simulink model "gm_hybrid_lht"  (R2019b)
settings: Solver=FixedStepDiscrete  StartTime=0.0  StopTime=inf  FixedStep=1/120e6  RelTol=1e-3
undefined symbols (not defined in the file or in its folder): bt, height, nTheta, width
libraries: hdlsllib x312, simulink x194, hdlmdlgenlib x7, dspsrcs4 x1
(part 9 of 13)

== system gm_hybrid_lht/Hybrid LHT/Hybrid LHT Kernel/Gradient Kernel System/Get Index and Fix Limits/GetShift1_instance21 ==
  Theta : Inport  OutDataTypeStr=uint8  PortDimensions=1  SampleTime=8.33333333333333e-09
  Add : Sum  Inputs=+  OutDataTypeStr=fixdt(0, ceil(log2(L+1)), 0)
  Constant : Constant  Value=U  VectorParams1D=off  OutDataTypeStr=fixdt(0,ceil(log2(max(U)+1)),0)  SampleTime=-1
  Relational Operator : RelationalOperator  OutDataTypeStr=boolean  RndMeth=Nearest
  Shift : Outport  VectorParamsAs1DForOutWhenUnconnected=off
  wires:
  Theta/1 -> Relational Operator/1
  Add/1 -> Shift/1
  Constant/1 -> Relational Operator/2
  Relational Operator/1 -> Add/1

== system gm_hybrid_lht/Hybrid LHT/Hybrid LHT Kernel/Gradient Kernel System/Get Index and Fix Limits/GetShift1_instance22 ==
  Theta : Inport  OutDataTypeStr=uint8  PortDimensions=1  SampleTime=8.33333333333333e-09
  Add : Sum  Inputs=+  OutDataTypeStr=fixdt(0, ceil(log2(L+1)), 0)
  Constant : Constant  Value=U  VectorParams1D=off  OutDataTypeStr=fixdt(0,ceil(log2(max(U)+1)),0)  SampleTime=-1
  Relational Operator : RelationalOperator  OutDataTypeStr=boolean  RndMeth=Nearest
  Shift : Outport  VectorParamsAs1DForOutWhenUnconnected=off
  wires:
  Theta/1 -> Relational Operator/1
  Add/1 -> Shift/1
  Constant/1 -> Relational Operator/2
  Relational Operator/1 -> Add/1

== system gm_hybrid_lht/Hybrid LHT/Hybrid LHT Kernel/Gradient Kernel System/Get Index and Fix Limits/GetShift1_instance23 ==
  Theta : Inport  OutDataTypeStr=uint8  PortDimensions=1  SampleTime=8.33333333333333e-09
  Add : Sum  Inputs=+  OutDataTypeStr=fixdt(0, ceil(log2(L+1)), 0)
  Constant : Constant  Value=U  VectorParams1D=off  OutDataTypeStr=fixdt(0,ceil(log2(max(U)+1)),0)  SampleTime=-1
  Relational Operator : RelationalOperator  OutDataTypeStr=boolean  RndMeth=Nearest
  Shift : Outport  VectorParamsAs1DForOutWhenUnconnected=off
  wires:
  Theta/1 -> Relational Operator/1
  Add/1 -> Shift/1
  Constant/1 -> Relational Operator/2
  Relational Operator/1 -> Add/1

== system gm_hybrid_lht/Hybrid LHT/Hybrid LHT Kernel/Gradient Kernel System/Get Index and Fix Limits/GetShift1_instance24 ==
  Theta : Inport  OutDataTypeStr=uint8  PortDimensions=1  SampleTime=8.33333333333333e-09
  Add : Sum  Inputs=+  OutDataTypeStr=fixdt(0, ceil(log2(L+1)), 0)
  Constant : Constant  Value=U  VectorParams1D=off  OutDataTypeStr=fixdt(0,ceil(log2(max(U)+1)),0)  SampleTime=-1
  Relational Operator : RelationalOperator  OutDataTypeStr=boolean  RndMeth=Nearest
  Shift : Outport  VectorParamsAs1DForOutWhenUnconnected=off
  wires:
  Theta/1 -> Relational Operator/1
  Add/1 -> Shift/1
  Constant/1 -> Relational Operator/2
  Relational Operator/1 -> Add/1

== system gm_hybrid_lht/Hybrid LHT/Hybrid LHT Kernel/Gradient Kernel System/Get Index and Fix Limits/GetShift1_instance25 ==
  Theta : Inport  OutDataTypeStr=uint8  PortDimensions=1  SampleTime=8.33333333333333e-09
  Add : Sum  Inputs=+  OutDataTypeStr=fixdt(0, ceil(log2(L+1)), 0)
  Constant : Constant  Value=U  VectorParams1D=off  OutDataTypeStr=fixdt(0,ceil(log2(max(U)+1)),0)  SampleTime=-1
  Relational Operator : RelationalOperator  OutDataTypeStr=boolean  RndMeth=Nearest
  Shift : Outport  VectorParamsAs1DForOutWhenUnconnected=off
  wires:
  Theta/1 -> Relational Operator/1
  Add/1 -> Shift/1
  Constant/1 -> Relational Operator/2
  Relational Operator/1 -> Add/1

== system gm_hybrid_lht/Hybrid LHT/Hybrid LHT Kernel/Gradient Kernel System/Get Index and Fix Limits/GetShift1_instance26 ==
  Theta : Inport  OutDataTypeStr=uint8  PortDimensions=1  SampleTime=8.33333333333333e-09
  Add : Sum  Inputs=+  OutDataTypeStr=fixdt(0, ceil(log2(L+1)), 0)
  Constant : Constant  Value=U  VectorParams1D=off  OutDataTypeStr=fixdt(0,ceil(log2(max(U)+1)),0)  SampleTime=-1
  Relational Operator : RelationalOperator  OutDataTypeStr=boolean  RndMeth=Nearest
  Shift : Outport  VectorParamsAs1DForOutWhenUnconnected=off
  wires:
  Theta/1 -> Relational Operator/1
  Add/1 -> Shift/1
  Constant/1 -> Relational Operator/2
  Relational Operator/1 -> Add/1

== system gm_hybrid_lht/Hybrid LHT/Hybrid LHT Kernel/Gradient Kernel System/Get Index and Fix Limits/GetShift1_instance27 ==
  Theta : Inport  OutDataTypeStr=uint8  PortDimensions=1  SampleTime=8.33333333333333e-09
  Add : Sum  Inputs=+  OutDataTypeStr=fixdt(0, ceil(log2(L+1)), 0)
  Constant : Constant  Value=U  VectorParams1D=off  OutDataTypeStr=fixdt(0,ceil(log2(max(U)+1)),0)  SampleTime=-1
  Relational Operator : RelationalOperator  OutDataTypeStr=boolean  RndMeth=Nearest
  Shift : Outport  VectorParamsAs1DForOutWhenUnconnected=off
  wires:
  Theta/1 -> Relational Operator/1
  Add/1 -> Shift/1
  Constant/1 -> Relational Operator/2
  Relational Operator/1 -> Add/1

== system gm_hybrid_lht/Hybrid LHT/Hybrid LHT Kernel/Gradient Kernel System/Get Index and Fix Limits/GetShift1_instance28 ==
  Theta : Inport  OutDataTypeStr=uint8  PortDimensions=1  SampleTime=8.33333333333333e-09
  Add : Sum  Inputs=+  OutDataTypeStr=fixdt(0, ceil(log2(L+1)), 0)
  Constant : Constant  Value=U  VectorParams1D=off  OutDataTypeStr=fixdt(0,ceil(log2(max(U)+1)),0)  SampleTime=-1
  Relational Operator : RelationalOperator  OutDataTypeStr=boolean  RndMeth=Nearest
  Shift : Outport  VectorParamsAs1DForOutWhenUnconnected=off
  wires:
  Theta/1 -> Relational Operator/1
  Add/1 -> Shift/1
  Constant/1 -> Relational Operator/2
  Relational Operator/1 -> Add/1

== system gm_hybrid_lht/Hybrid LHT/Hybrid LHT Kernel/Gradient Kernel System/Get Index and Fix Limits/GetShift1_instance29 ==
  Theta : Inport  OutDataTypeStr=uint8  PortDimensions=1  SampleTime=8.33333333333333e-09
  Add : Sum  Inputs=+  OutDataTypeStr=fixdt(0, ceil(log2(L+1)), 0)
  Constant : Constant  Value=U  VectorParams1D=off  OutDataTypeStr=fixdt(0,ceil(log2(max(U)+1)),0)  SampleTime=-1
  Relational Operator : RelationalOperator  OutDataTypeStr=boolean  RndMeth=Nearest
  Shift : Outport  VectorParamsAs1DForOutWhenUnconnected=off
  wires:
  Theta/1 -> Relational Operator/1
  Add/1 -> Shift/1
  Constant/1 -> Relational Operator/2
  Relational Operator/1 -> Add/1

== system gm_hybrid_lht/Hybrid LHT/Hybrid LHT Kernel/Gradient Kernel System/Get Index and Fix Limits/GetShift1_instance3 ==
  Theta : Inport  OutDataTypeStr=uint8  PortDimensions=1  SampleTime=8.33333333333333e-09
  Add : Sum  Inputs=+  OutDataTypeStr=fixdt(0, ceil(log2(L+1)), 0)
  Constant : Constant  Value=U  VectorParams1D=off  OutDataTypeStr=fixdt(0,ceil(log2(max(U)+1)),0)  SampleTime=-1
  Relational Operator : RelationalOperator  OutDataTypeStr=boolean  RndMeth=Nearest
  Shift : Outport  VectorParamsAs1DForOutWhenUnconnected=off
  wires:
  Theta/1 -> Relational Operator/1
  Add/1 -> Shift/1
  Constant/1 -> Relational Operator/2
  Relational Operator/1 -> Add/1

== system gm_hybrid_lht/Hybrid LHT/Hybrid LHT Kernel/Gradient Kernel System/Get Index and Fix Limits/GetShift1_instance30 ==
  Theta : Inport  OutDataTypeStr=uint8  PortDimensions=1  SampleTime=8.33333333333333e-09
  Add : Sum  Inputs=+  OutDataTypeStr=fixdt(0, ceil(log2(L+1)), 0)
  Constant : Constant  Value=U  VectorParams1D=off  OutDataTypeStr=fixdt(0,ceil(log2(max(U)+1)),0)  SampleTime=-1
  Relational Operator : RelationalOperator  OutDataTypeStr=boolean  RndMeth=Nearest
  Shift : Outport  VectorParamsAs1DForOutWhenUnconnected=off
  wires:
  Theta/1 -> Relational Operator/1
  Add/1 -> Shift/1
  Constant/1 -> Relational Operator/2
  Relational Operator/1 -> Add/1

== system gm_hybrid_lht/Hybrid LHT/Hybrid LHT Kernel/Gradient Kernel System/Get Index and Fix Limits/GetShift1_instance31 ==
  Theta : Inport  OutDataTypeStr=uint8  PortDimensions=1  SampleTime=8.33333333333333e-09
  Add : Sum  Inputs=+  OutDataTypeStr=fixdt(0, ceil(log2(L+1)), 0)
  Constant : Constant  Value=U  VectorParams1D=off  OutDataTypeStr=fixdt(0,ceil(log2(max(U)+1)),0)  SampleTime=-1
  Relational Operator : RelationalOperator  OutDataTypeStr=boolean  RndMeth=Nearest
  Shift : Outport  VectorParamsAs1DForOutWhenUnconnected=off
  wires:
  Theta/1 -> Relational Operator/1
  Add/1 -> Shift/1
  Constant/1 -> Relational Operator/2
  Relational Operator/1 -> Add/1

== system gm_hybrid_lht/Hybrid LHT/Hybrid LHT Kernel/Gradient Kernel System/Get Index and Fix Limits/GetShift1_instance32 ==
  Theta : Inport  OutDataTypeStr=uint8  PortDimensions=1  SampleTime=8.33333333333333e-09
  Add : Sum  Inputs=+  OutDataTypeStr=fixdt(0, ceil(log2(L+1)), 0)
  Constant : Constant  Value=U  VectorParams1D=off  OutDataTypeStr=fixdt(0,ceil(log2(max(U)+1)),0)  SampleTime=-1
  Relational Operator : RelationalOperator  OutDataTypeStr=boolean  RndMeth=Nearest
  Shift : Outport  VectorParamsAs1DForOutWhenUnconnected=off
  wires:
  Theta/1 -> Relational Operator/1
  Add/1 -> Shift/1
  Constant/1 -> Relational Operator/2
  Relational Operator/1 -> Add/1

== system gm_hybrid_lht/Hybrid LHT/Hybrid LHT Kernel/Gradient Kernel System/Get Index and Fix Limits/GetShift1_instance33 ==
  Theta : Inport  OutDataTypeStr=uint8  PortDimensions=1  SampleTime=8.33333333333333e-09
  Add : Sum  Inputs=+  OutDataTypeStr=fixdt(0, ceil(log2(L+1)), 0)
  Constant : Constant  Value=U  VectorParams1D=off  OutDataTypeStr=fixdt(0,ceil(log2(max(U)+1)),0)  SampleTime=-1
  Relational Operator : RelationalOperator  OutDataTypeStr=boolean  RndMeth=Nearest
  Shift : Outport  VectorParamsAs1DForOutWhenUnconnected=off
  wires:
  Theta/1 -> Relational Operator/1
  Add/1 -> Shift/1
  Constant/1 -> Relational Operator/2
  Relational Operator/1 -> Add/1

== system gm_hybrid_lht/Hybrid LHT/Hybrid LHT Kernel/Gradient Kernel System/Get Index and Fix Limits/GetShift1_instance34 ==
  Theta : Inport  OutDataTypeStr=uint8  PortDimensions=1  SampleTime=8.33333333333333e-09
  Add : Sum  Inputs=+  OutDataTypeStr=fixdt(0, ceil(log2(L+1)), 0)
  Constant : Constant  Value=U  VectorParams1D=off  OutDataTypeStr=fixdt(0,ceil(log2(max(U)+1)),0)  SampleTime=-1
  Relational Operator : RelationalOperator  OutDataTypeStr=boolean  RndMeth=Nearest
  Shift : Outport  VectorParamsAs1DForOutWhenUnconnected=off
  wires:
  Theta/1 -> Relational Operator/1
  Add/1 -> Shift/1
  Constant/1 -> Relational Operator/2
  Relational Operator/1 -> Add/1

== system gm_hybrid_lht/Hybrid LHT/Hybrid LHT Kernel/Gradient Kernel System/Get Index and Fix Limits/GetShift1_instance35 ==
  Theta : Inport  OutDataTypeStr=uint8  PortDimensions=1  SampleTime=8.33333333333333e-09
  Add : Sum  Inputs=+  OutDataTypeStr=fixdt(0, ceil(log2(L+1)), 0)
  Constant : Constant  Value=U  VectorParams1D=off  OutDataTypeStr=fixdt(0,ceil(log2(max(U)+1)),0)  SampleTime=-1
  Relational Operator : RelationalOperator  OutDataTypeStr=boolean  RndMeth=Nearest
  Shift : Outport  VectorParamsAs1DForOutWhenUnconnected=off
  wires:
  Theta/1 -> Relational Operator/1
  Add/1 -> Shift/1
  Constant/1 -> Relational Operator/2
  Relational Operator/1 -> Add/1

== system gm_hybrid_lht/Hybrid LHT/Hybrid LHT Kernel/Gradient Kernel System/Get Index and Fix Limits/GetShift1_instance36 ==
  Theta : Inport  OutDataTypeStr=uint8  PortDimensions=1  SampleTime=8.33333333333333e-09
  Add : Sum  Inputs=+  OutDataTypeStr=fixdt(0, ceil(log2(L+1)), 0)
  Constant : Constant  Value=U  VectorParams1D=off  OutDataTypeStr=fixdt(0,ceil(log2(max(U)+1)),0)  SampleTime=-1
  Relational Operator : RelationalOperator  OutDataTypeStr=boolean  RndMeth=Nearest
  Shift : Outport  VectorParamsAs1DForOutWhenUnconnected=off
  wires:
  Theta/1 -> Relational Operator/1
  Add/1 -> Shift/1
  Constant/1 -> Relational Operator/2
  Relational Operator/1 -> Add/1

== system gm_hybrid_lht/Hybrid LHT/Hybrid LHT Kernel/Gradient Kernel System/Get Index and Fix Limits/GetShift1_instance37 ==
  Theta : Inport  OutDataTypeStr=uint8  PortDimensions=1  SampleTime=8.33333333333333e-09
  Add : Sum  Inputs=+  OutDataTypeStr=fixdt(0, ceil(log2(L+1)), 0)
  Constant : Constant  Value=U  VectorParams1D=off  OutDataTypeStr=fixdt(0,ceil(log2(max(U)+1)),0)  SampleTime=-1
  Relational Operator : RelationalOperator  OutDataTypeStr=boolean  RndMeth=Nearest
  Shift : Outport  VectorParamsAs1DForOutWhenUnconnected=off
  wires:
  Theta/1 -> Relational Operator/1
  Add/1 -> Shift/1
  Constant/1 -> Relational Operator/2
  Relational Operator/1 -> Add/1

== system gm_hybrid_lht/Hybrid LHT/Hybrid LHT Kernel/Gradient Kernel System/Get Index and Fix Limits/GetShift1_instance38 ==
  Theta : Inport  OutDataTypeStr=uint8  PortDimensions=1  SampleTime=8.33333333333333e-09
  Add : Sum  Inputs=+  OutDataTypeStr=fixdt(0, ceil(log2(L+1)), 0)
  Constant : Constant  Value=U  VectorParams1D=off  OutDataTypeStr=fixdt(0,ceil(log2(max(U)+1)),0)  SampleTime=-1
  Relational Operator : RelationalOperator  OutDataTypeStr=boolean  RndMeth=Nearest
  Shift : Outport  VectorParamsAs1DForOutWhenUnconnected=off
  wires:
  Theta/1 -> Relational Operator/1
  Add/1 -> Shift/1
  Constant/1 -> Relational Operator/2
  Relational Operator/1 -> Add/1

== system gm_hybrid_lht/Hybrid LHT/Hybrid LHT Kernel/Gradient Kernel System/Get Index and Fix Limits/GetShift1_instance39 ==
  Theta : Inport  OutDataTypeStr=uint8  PortDimensions=1  SampleTime=8.33333333333333e-09
  Add : Sum  Inputs=+  OutDataTypeStr=fixdt(0, ceil(log2(L+1)), 0)
  Constant : Constant  Value=U  VectorParams1D=off  OutDataTypeStr=fixdt(0,ceil(log2(max(U)+1)),0)  SampleTime=-1
  Relational Operator : RelationalOperator  OutDataTypeStr=boolean  RndMeth=Nearest
  Shift : Outport  VectorParamsAs1DForOutWhenUnconnected=off
  wires:
  Theta/1 -> Relational Operator/1
  Add/1 -> Shift/1
  Constant/1 -> Relational Operator/2
  Relational Operator/1 -> Add/1

== system gm_hybrid_lht/Hybrid LHT/Hybrid LHT Kernel/Gradient Kernel System/Get Index and Fix Limits/GetShift1_instance4 ==
  Theta : Inport  OutDataTypeStr=uint8  PortDimensions=1  SampleTime=8.33333333333333e-09
  Add : Sum  Inputs=+  OutDataTypeStr=fixdt(0, ceil(log2(L+1)), 0)
  Constant : Constant  Value=U  VectorParams1D=off  OutDataTypeStr=fixdt(0,ceil(log2(max(U)+1)),0)  SampleTime=-1
  Relational Operator : RelationalOperator  OutDataTypeStr=boolean  RndMeth=Nearest
  Shift : Outport  VectorParamsAs1DForOutWhenUnconnected=off
  wires:
  Theta/1 -> Relational Operator/1
  Add/1 -> Shift/1
  Constant/1 -> Relational Operator/2
  Relational Operator/1 -> Add/1

== system gm_hybrid_lht/Hybrid LHT/Hybrid LHT Kernel/Gradient Kernel System/Get Index and Fix Limits/GetShift1_instance40 ==
  Theta : Inport  OutDataTypeStr=uint8  PortDimensions=1  SampleTime=8.33333333333333e-09
  Add : Sum  Inputs=+  OutDataTypeStr=fixdt(0, ceil(log2(L+1)), 0)
  Constant : Constant  Value=U  VectorParams1D=off  OutDataTypeStr=fixdt(0,ceil(log2(max(U)+1)),0)  SampleTime=-1
  Relational Operator : RelationalOperator  OutDataTypeStr=boolean  RndMeth=Nearest
  Shift : Outport  VectorParamsAs1DForOutWhenUnconnected=off
  wires:
  Theta/1 -> Relational Operator/1
  Add/1 -> Shift/1
  Constant/1 -> Relational Operator/2
  Relational Operator/1 -> Add/1

== system gm_hybrid_lht/Hybrid LHT/Hybrid LHT Kernel/Gradient Kernel System/Get Index and Fix Limits/GetShift1_instance41 ==
  Theta : Inport  OutDataTypeStr=uint8  PortDimensions=1  SampleTime=8.33333333333333e-09
  Add : Sum  Inputs=+  OutDataTypeStr=fixdt(0, ceil(log2(L+1)), 0)
  Constant : Constant  Value=U  VectorParams1D=off  OutDataTypeStr=fixdt(0,ceil(log2(max(U)+1)),0)  SampleTime=-1
  Relational Operator : RelationalOperator  OutDataTypeStr=boolean  RndMeth=Nearest
  Shift : Outport  VectorParamsAs1DForOutWhenUnconnected=off
  wires:
  Theta/1 -> Relational Operator/1
  Add/1 -> Shift/1
  Constant/1 -> Relational Operator/2
  Relational Operator/1 -> Add/1

== system gm_hybrid_lht/Hybrid LHT/Hybrid LHT Kernel/Gradient Kernel System/Get Index and Fix Limits/GetShift1_instance42 ==
  Theta : Inport  OutDataTypeStr=uint8  PortDimensions=1  SampleTime=8.33333333333333e-09
  Add : Sum  Inputs=+  OutDataTypeStr=fixdt(0, ceil(log2(L+1)), 0)
  Constant : Constant  Value=U  VectorParams1D=off  OutDataTypeStr=fixdt(0,ceil(log2(max(U)+1)),0)  SampleTime=-1
  Relational Operator : RelationalOperator  OutDataTypeStr=boolean  RndMeth=Nearest
  Shift : Outport  VectorParamsAs1DForOutWhenUnconnected=off
  wires:
  Theta/1 -> Relational Operator/1
  Add/1 -> Shift/1
  Constant/1 -> Relational Operator/2
  Relational Operator/1 -> Add/1

== system gm_hybrid_lht/Hybrid LHT/Hybrid LHT Kernel/Gradient Kernel System/Get Index and Fix Limits/GetShift1_instance43 ==
  Theta : Inport  OutDataTypeStr=uint8  PortDimensions=1  SampleTime=8.33333333333333e-09
  Add : Sum  Inputs=+  OutDataTypeStr=fixdt(0, ceil(log2(L+1)), 0)
  Constant : Constant  Value=U  VectorParams1D=off  OutDataTypeStr=fixdt(0,ceil(log2(max(U)+1)),0)  SampleTime=-1
  Relational Operator : RelationalOperator  OutDataTypeStr=boolean  RndMeth=Nearest
  Shift : Outport  VectorParamsAs1DForOutWhenUnconnected=off
  wires:
  Theta/1 -> Relational Operator/1
  Add/1 -> Shift/1
  Constant/1 -> Relational Operator/2
  Relational Operator/1 -> Add/1

== system gm_hybrid_lht/Hybrid LHT/Hybrid LHT Kernel/Gradient Kernel System/Get Index and Fix Limits/GetShift1_instance44 ==
  Theta : Inport  OutDataTypeStr=uint8  PortDimensions=1  SampleTime=8.33333333333333e-09
  Add : Sum  Inputs=+  OutDataTypeStr=fixdt(0, ceil(log2(L+1)), 0)
  Constant : Constant  Value=U  VectorParams1D=off  OutDataTypeStr=fixdt(0,ceil(log2(max(U)+1)),0)  SampleTime=-1
  Relational Operator : RelationalOperator  OutDataTypeStr=boolean  RndMeth=Nearest
  Shift : Outport  VectorParamsAs1DForOutWhenUnconnected=off
  wires:
  Theta/1 -> Relational Operator/1
  Add/1 -> Shift/1
  Constant/1 -> Relational Operator/2
  Relational Operator/1 -> Add/1

== system gm_hybrid_lht/Hybrid LHT/Hybrid LHT Kernel/Gradient Kernel System/Get Index and Fix Limits/GetShift1_instance45 ==
  Theta : Inport  OutDataTypeStr=uint8  PortDimensions=1  SampleTime=8.33333333333333e-09
  Add : Sum  Inputs=+  OutDataTypeStr=fixdt(0, ceil(log2(L+1)), 0)
  Constant : Constant  Value=U  VectorParams1D=off  OutDataTypeStr=fixdt(0,ceil(log2(max(U)+1)),0)  SampleTime=-1
  Relational Operator : RelationalOperator  OutDataTypeStr=boolean  RndMeth=Nearest
  Shift : Outport  VectorParamsAs1DForOutWhenUnconnected=off
  wires:
  Theta/1 -> Relational Operator/1
  Add/1 -> Shift/1
  Constant/1 -> Relational Operator/2
  Relational Operator/1 -> Add/1

== system gm_hybrid_lht/Hybrid LHT/Hybrid LHT Kernel/Gradient Kernel System/Get Index and Fix Limits/GetShift1_instance46 ==
  Theta : Inport  OutDataTypeStr=uint8  PortDimensions=1  SampleTime=8.33333333333333e-09
  Add : Sum  Inputs=+  OutDataTypeStr=fixdt(0, ceil(log2(L+1)), 0)
  Constant : Constant  Value=U  VectorParams1D=off  OutDataTypeStr=fixdt(0,ceil(log2(max(U)+1)),0)  SampleTime=-1
  Relational Operator : RelationalOperator  OutDataTypeStr=boolean  RndMeth=Nearest
  Shift : Outport  VectorParamsAs1DForOutWhenUnconnected=off
  wires:
  Theta/1 -> Relational Operator/1
  Add/1 -> Shift/1
  Constant/1 -> Relational Operator/2
  Relational Operator/1 -> Add/1

== system gm_hybrid_lht/Hybrid LHT/Hybrid LHT Kernel/Gradient Kernel System/Get Index and Fix Limits/GetShift1_instance47 ==
  Theta : Inport  OutDataTypeStr=uint8  PortDimensions=1  SampleTime=8.33333333333333e-09
  Add : Sum  Inputs=+  OutDataTypeStr=fixdt(0, ceil(log2(L+1)), 0)
  Constant : Constant  Value=U  VectorParams1D=off  OutDataTypeStr=fixdt(0,ceil(log2(max(U)+1)),0)  SampleTime=-1
  Relational Operator : RelationalOperator  OutDataTypeStr=boolean  RndMeth=Nearest
  Shift : Outport  VectorParamsAs1DForOutWhenUnconnected=off
  wires:
  Theta/1 -> Relational Operator/1
  Add/1 -> Shift/1
  Constant/1 -> Relational Operator/2
  Relational Operator/1 -> Add/1

== system gm_hybrid_lht/Hybrid LHT/Hybrid LHT Kernel/Gradient Kernel System/Get Index and Fix Limits/GetShift1_instance48 ==
  Theta : Inport  OutDataTypeStr=uint8  PortDimensions=1  SampleTime=8.33333333333333e-09
  Add : Sum  Inputs=+  OutDataTypeStr=fixdt(0, ceil(log2(L+1)), 0)
  Constant : Constant  Value=U  VectorParams1D=off  OutDataTypeStr=fixdt(0,ceil(log2(max(U)+1)),0)  SampleTime=-1
  Relational Operator : RelationalOperator  OutDataTypeStr=boolean  RndMeth=Nearest
  Shift : Outport  VectorParamsAs1DForOutWhenUnconnected=off
  wires:
  Theta/1 -> Relational Operator/1
  Add/1 -> Shift/1
  Constant/1 -> Relational Operator/2
  Relational Operator/1 -> Add/1

== system gm_hybrid_lht/Hybrid LHT/Hybrid LHT Kernel/Gradient Kernel System/Get Index and Fix Limits/GetShift1_instance49 ==
  Theta : Inport  OutDataTypeStr=uint8  PortDimensions=1  SampleTime=8.33333333333333e-09
  Add : Sum  Inputs=+  OutDataTypeStr=fixdt(0, ceil(log2(L+1)), 0)
  Constant : Constant  Value=U  VectorParams1D=off  OutDataTypeStr=fixdt(0,ceil(log2(max(U)+1)),0)  SampleTime=-1
  Relational Operator : RelationalOperator  OutDataTypeStr=boolean  RndMeth=Nearest
  Shift : Outport  VectorParamsAs1DForOutWhenUnconnected=off
  wires:
  Theta/1 -> Relational Operator/1
  Add/1 -> Shift/1
  Constant/1 -> Relational Operator/2
  Relational Operator/1 -> Add/1

== system gm_hybrid_lht/Hybrid LHT/Hybrid LHT Kernel/Gradient Kernel System/Get Index and Fix Limits/GetShift1_instance5 ==
  Theta : Inport  OutDataTypeStr=uint8  PortDimensions=1  SampleTime=8.33333333333333e-09
  Add : Sum  Inputs=+  OutDataTypeStr=fixdt(0, ceil(log2(L+1)), 0)
  Constant : Constant  Value=U  VectorParams1D=off  OutDataTypeStr=fixdt(0,ceil(log2(max(U)+1)),0)  SampleTime=-1
  Relational Operator : RelationalOperator  OutDataTypeStr=boolean  RndMeth=Nearest
  Shift : Outport  VectorParamsAs1DForOutWhenUnconnected=off
  wires:
  Theta/1 -> Relational Operator/1
  Add/1 -> Shift/1
  Constant/1 -> Relational Operator/2
  Relational Operator/1 -> Add/1

== system gm_hybrid_lht/Hybrid LHT/Hybrid LHT Kernel/Gradient Kernel System/Get Index and Fix Limits/GetShift1_instance50 ==
  Theta : Inport  OutDataTypeStr=uint8  PortDimensions=1  SampleTime=8.33333333333333e-09
  Add : Sum  Inputs=+  OutDataTypeStr=fixdt(0, ceil(log2(L+1)), 0)
  Constant : Constant  Value=U  VectorParams1D=off  OutDataTypeStr=fixdt(0,ceil(log2(max(U)+1)),0)  SampleTime=-1
  Relational Operator : RelationalOperator  OutDataTypeStr=boolean  RndMeth=Nearest
  Shift : Outport  VectorParamsAs1DForOutWhenUnconnected=off
  wires:
  Theta/1 -> Relational Operator/1
  Add/1 -> Shift/1
  Constant/1 -> Relational Operator/2
  Relational Operator/1 -> Add/1

== system gm_hybrid_lht/Hybrid LHT/Hybrid LHT Kernel/Gradient Kernel System/Get Index and Fix Limits/GetShift1_instance51 ==
  Theta : Inport  OutDataTypeStr=uint8  PortDimensions=1  SampleTime=8.33333333333333e-09
  Add : Sum  Inputs=+  OutDataTypeStr=fixdt(0, ceil(log2(L+1)), 0)
  Constant : Constant  Value=U  VectorParams1D=off  OutDataTypeStr=fixdt(0,ceil(log2(max(U)+1)),0)  SampleTime=-1
  Relational Operator : RelationalOperator  OutDataTypeStr=boolean  RndMeth=Nearest
  Shift : Outport  VectorParamsAs1DForOutWhenUnconnected=off
  wires:
  Theta/1 -> Relational Operator/1
  Add/1 -> Shift/1
  Constant/1 -> Relational Operator/2
  Relational Operator/1 -> Add/1

== system gm_hybrid_lht/Hybrid LHT/Hybrid LHT Kernel/Gradient Kernel System/Get Index and Fix Limits/GetShift1_instance52 ==
  Theta : Inport  OutDataTypeStr=uint8  PortDimensions=1  SampleTime=8.33333333333333e-09
  Add : Sum  Inputs=+  OutDataTypeStr=fixdt(0, ceil(log2(L+1)), 0)
  Constant : Constant  Value=U  VectorParams1D=off  OutDataTypeStr=fixdt(0,ceil(log2(max(U)+1)),0)  SampleTime=-1
  Relational Operator : RelationalOperator  OutDataTypeStr=boolean  RndMeth=Nearest
  Shift : Outport  VectorParamsAs1DForOutWhenUnconnected=off
  wires:
  Theta/1 -> Relational Operator/1
  Add/1 -> Shift/1
  Constant/1 -> Relational Operator/2
  Relational Operator/1 -> Add/1

== system gm_hybrid_lht/Hybrid LHT/Hybrid LHT Kernel/Gradient Kernel System/Get Index and Fix Limits/GetShift1_instance53 ==
  Theta : Inport  OutDataTypeStr=uint8  PortDimensions=1  SampleTime=8.33333333333333e-09
  Add : Sum  Inputs=+  OutDataTypeStr=fixdt(0, ceil(log2(L+1)), 0)
  Constant : Constant  Value=U  VectorParams1D=off  OutDataTypeStr=fixdt(0,ceil(log2(max(U)+1)),0)  SampleTime=-1
  Relational Operator : RelationalOperator  OutDataTypeStr=boolean  RndMeth=Nearest
  Shift : Outport  VectorParamsAs1DForOutWhenUnconnected=off
  wires:
  Theta/1 -> Relational Operator/1
  Add/1 -> Shift/1
  Constant/1 -> Relational Operator/2
  Relational Operator/1 -> Add/1

== system gm_hybrid_lht/Hybrid LHT/Hybrid LHT Kernel/Gradient Kernel System/Get Index and Fix Limits/GetShift1_instance54 ==
  Theta : Inport  OutDataTypeStr=uint8  PortDimensions=1  SampleTime=8.33333333333333e-09
  Add : Sum  Inputs=+  OutDataTypeStr=fixdt(0, ceil(log2(L+1)), 0)
  Constant : Constant  Value=U  VectorParams1D=off  OutDataTypeStr=fixdt(0,ceil(log2(max(U)+1)),0)  SampleTime=-1
  Relational Operator : RelationalOperator  OutDataTypeStr=boolean  RndMeth=Nearest
  Shift : Outport  VectorParamsAs1DForOutWhenUnconnected=off
  wires:
  Theta/1 -> Relational Operator/1
  Add/1 -> Shift/1
  Constant/1 -> Relational Operator/2
  Relational Operator/1 -> Add/1

== system gm_hybrid_lht/Hybrid LHT/Hybrid LHT Kernel/Gradient Kernel System/Get Index and Fix Limits/GetShift1_instance55 ==
  Theta : Inport  OutDataTypeStr=uint8  PortDimensions=1  SampleTime=8.33333333333333e-09
  Add : Sum  Inputs=+  OutDataTypeStr=fixdt(0, ceil(log2(L+1)), 0)
  Constant : Constant  Value=U  VectorParams1D=off  OutDataTypeStr=fixdt(0,ceil(log2(max(U)+1)),0)  SampleTime=-1
  Relational Operator : RelationalOperator  OutDataTypeStr=boolean  RndMeth=Nearest
  Shift : Outport  VectorParamsAs1DForOutWhenUnconnected=off
  wires:
  Theta/1 -> Relational Operator/1
  Add/1 -> Shift/1
  Constant/1 -> Relational Operator/2
  Relational Operator/1 -> Add/1

== system gm_hybrid_lht/Hybrid LHT/Hybrid LHT Kernel/Gradient Kernel System/Get Index and Fix Limits/GetShift1_instance56 ==
  Theta : Inport  OutDataTypeStr=uint8  PortDimensions=1  SampleTime=8.33333333333333e-09
  Add : Sum  Inputs=+  OutDataTypeStr=fixdt(0, ceil(log2(L+1)), 0)
  Constant : Constant  Value=U  VectorParams1D=off  OutDataTypeStr=fixdt(0,ceil(log2(max(U)+1)),0)  SampleTime=-1
  Relational Operator : RelationalOperator  OutDataTypeStr=boolean  RndMeth=Nearest
  Shift : Outport  VectorParamsAs1DForOutWhenUnconnected=off
  wires:
  Theta/1 -> Relational Operator/1
  Add/1 -> Shift/1
  Constant/1 -> Relational Operator/2
  Relational Operator/1 -> Add/1

== system gm_hybrid_lht/Hybrid LHT/Hybrid LHT Kernel/Gradient Kernel System/Get Index and Fix Limits/GetShift1_instance57 ==
  Theta : Inport  OutDataTypeStr=uint8  PortDimensions=1  SampleTime=8.33333333333333e-09
  Add : Sum  Inputs=+  OutDataTypeStr=fixdt(0, ceil(log2(L+1)), 0)
  Constant : Constant  Value=U  VectorParams1D=off  OutDataTypeStr=fixdt(0,ceil(log2(max(U)+1)),0)  SampleTime=-1
  Relational Operator : RelationalOperator  OutDataTypeStr=boolean  RndMeth=Nearest
  Shift : Outport  VectorParamsAs1DForOutWhenUnconnected=off
  wires:
  Theta/1 -> Relational Operator/1
  Add/1 -> Shift/1
  Constant/1 -> Relational Operator/2
  Relational Operator/1 -> Add/1

== system gm_hybrid_lht/Hybrid LHT/Hybrid LHT Kernel/Gradient Kernel System/Get Index and Fix Limits/GetShift1_instance58 ==
  Theta : Inport  OutDataTypeStr=uint8  PortDimensions=1  SampleTime=8.33333333333333e-09
  Add : Sum  Inputs=+  OutDataTypeStr=fixdt(0, ceil(log2(L+1)), 0)
  Constant : Constant  Value=U  VectorParams1D=off  OutDataTypeStr=fixdt(0,ceil(log2(max(U)+1)),0)  SampleTime=-1
  Relational Operator : RelationalOperator  OutDataTypeStr=boolean  RndMeth=Nearest
  Shift : Outport  VectorParamsAs1DForOutWhenUnconnected=off
  wires:
  Theta/1 -> Relational Operator/1
  Add/1 -> Shift/1
  Constant/1 -> Relational Operator/2
  Relational Operator/1 -> Add/1

== system gm_hybrid_lht/Hybrid LHT/Hybrid LHT Kernel/Gradient Kernel System/Get Index and Fix Limits/GetShift1_instance59 ==
  Theta : Inport  OutDataTypeStr=uint8  PortDimensions=1  SampleTime=8.33333333333333e-09
  Add : Sum  Inputs=+  OutDataTypeStr=fixdt(0, ceil(log2(L+1)), 0)
  Constant : Constant  Value=U  VectorParams1D=off  OutDataTypeStr=fixdt(0,ceil(log2(max(U)+1)),0)  SampleTime=-1
  Relational Operator : RelationalOperator  OutDataTypeStr=boolean  RndMeth=Nearest
  Shift : Outport  VectorParamsAs1DForOutWhenUnconnected=off
  wires:
  Theta/1 -> Relational Operator/1
  Add/1 -> Shift/1
  Constant/1 -> Relational Operator/2
  Relational Operator/1 -> Add/1

== system gm_hybrid_lht/Hybrid LHT/Hybrid LHT Kernel/Gradient Kernel System/Get Index and Fix Limits/GetShift1_instance6 ==
  Theta : Inport  OutDataTypeStr=uint8  PortDimensions=1  SampleTime=8.33333333333333e-09
  Add : Sum  Inputs=+  OutDataTypeStr=fixdt(0, ceil(log2(L+1)), 0)
  Constant : Constant  Value=U  VectorParams1D=off  OutDataTypeStr=fixdt(0,ceil(log2(max(U)+1)),0)  SampleTime=-1
  Relational Operator : RelationalOperator  OutDataTypeStr=boolean  RndMeth=Nearest
  Shift : Outport  VectorParamsAs1DForOutWhenUnconnected=off
  wires:
  Theta/1 -> Relational Operator/1
  Add/1 -> Shift/1
  Constant/1 -> Relational Operator/2
  Relational Operator/1 -> Add/1

== system gm_hybrid_lht/Hybrid LHT/Hybrid LHT Kernel/Gradient Kernel System/Get Index and Fix Limits/GetShift1_instance60 ==
  Theta : Inport  OutDataTypeStr=uint8  PortDimensions=1  SampleTime=8.33333333333333e-09
  Add : Sum  Inputs=+  OutDataTypeStr=fixdt(0, ceil(log2(L+1)), 0)
  Constant : Constant  Value=U  VectorParams1D=off  OutDataTypeStr=fixdt(0,ceil(log2(max(U)+1)),0)  SampleTime=-1
  Relational Operator : RelationalOperator  OutDataTypeStr=boolean  RndMeth=Nearest
  Shift : Outport  VectorParamsAs1DForOutWhenUnconnected=off
  wires:
  Theta/1 -> Relational Operator/1
  Add/1 -> Shift/1
  Constant/1 -> Relational Operator/2
  Relational Operator/1 -> Add/1

== system gm_hybrid_lht/Hybrid LHT/Hybrid LHT Kernel/Gradient Kernel System/Get Index and Fix Limits/GetShift1_instance7 ==
  Theta : Inport  OutDataTypeStr=uint8  PortDimensions=1  SampleTime=8.33333333333333e-09
  Add : Sum  Inputs=+  OutDataTypeStr=fixdt(0, ceil(log2(L+1)), 0)
  Constant : Constant  Value=U  VectorParams1D=off  OutDataTypeStr=fixdt(0,ceil(log2(max(U)+1)),0)  SampleTime=-1
  Relational Operator : RelationalOperator  OutDataTypeStr=boolean  RndMeth=Nearest
  Shift : Outport  VectorParamsAs1DForOutWhenUnconnected=off
  wires:
  Theta/1 -> Relational Operator/1
  Add/1 -> Shift/1
  Constant/1 -> Relational Operator/2
  Relational Operator/1 -> Add/1

== system gm_hybrid_lht/Hybrid LHT/Hybrid LHT Kernel/Gradient Kernel System/Get Index and Fix Limits/GetShift1_instance8 ==
  Theta : Inport  OutDataTypeStr=uint8  PortDimensions=1  SampleTime=8.33333333333333e-09
  Add : Sum  Inputs=+  OutDataTypeStr=fixdt(0, ceil(log2(L+1)), 0)
  Constant : Constant  Value=U  VectorParams1D=off  OutDataTypeStr=fixdt(0,ceil(log2(max(U)+1)),0)  SampleTime=-1
  Relational Operator : RelationalOperator  OutDataTypeStr=boolean  RndMeth=Nearest
  Shift : Outport  VectorParamsAs1DForOutWhenUnconnected=off
  wires:
  Theta/1 -> Relational Operator/1
  Add/1 -> Shift/1
  Constant/1 -> Relational Operator/2
  Relational Operator/1 -> Add/1

== system gm_hybrid_lht/Hybrid LHT/Hybrid LHT Kernel/Gradient Kernel System/Get Index and Fix Limits/GetShift1_instance9 ==
  Theta : Inport  OutDataTypeStr=uint8  PortDimensions=1  SampleTime=8.33333333333333e-09
  Add : Sum  Inputs=+  OutDataTypeStr=fixdt(0, ceil(log2(L+1)), 0)
  Constant : Constant  Value=U  VectorParams1D=off  OutDataTypeStr=fixdt(0,ceil(log2(max(U)+1)),0)  SampleTime=-1
  Relational Operator : RelationalOperator  OutDataTypeStr=boolean  RndMeth=Nearest
  Shift : Outport  VectorParamsAs1DForOutWhenUnconnected=off
  wires:
  Theta/1 -> Relational Operator/1
  Add/1 -> Shift/1
  Constant/1 -> Relational Operator/2
  Relational Operator/1 -> Add/1

== system gm_hybrid_lht/Hybrid LHT/Hybrid LHT Kernel/Gradient Kernel System/Hough Kernel/Hough Kernel ==
  X : Inport  OutDataTypeStr=fixdt(1, 9, 0)  PortDimensions=1  SampleTime=8.33333333333333e-09
  Y : Inport  Port=2  OutDataTypeStr=fixdt(1, 9, 0)  PortDimensions=[1 180]  SampleTime=8.33333333333333e-09
  Index : Inport  Port=3  OutDataTypeStr=uint8  PortDimensions=[1 60]  SampleTime=8.33333333333333e-09
  Add : Sum  AccumDataTypeStr=fixdt(1, 11, 0)  OutDataTypeStr=fixdt(1, 10, 0)  RndMeth=Round  SampleTime=8.33333333333333e-09
  CosineROM : Constant  Value=[1 0.9998779296875 0.9993896484375 0.9986572265625 0.99755859375 0.9962158203125 0.9945068359375 0.9925537109375 0.99029541015625 0.9876708984375 0.98480224609375 0.98162841796875 0.9781494140625 0.974365234375 0.97027587890625 0.9659423828125 0.96124267578125 0.956298828125 0.9510498046875 0.94549560546875 0.939697265625 0.93359375 0.92718505859375 0.9205322265625 0.91357421875 0.90631103515625 0.8988037109375 0.8909912109375 0.8829345703125 0.8746337890625 0.86602783203125 0.857177734375 0.8480224609375 0.83868408203125 0.82904052734375 0.81915283203125 0.80902099609375 0.79864501953125 0.78802490234375 0.77716064453125 0.76605224609375 0.75469970703125 0.7431640625 0.7313232421875 0.7193603515625 0.70709228515625 0.69464111328125 0.6820068359375 0.66912841796875 0.65606689453125 0.64276123046875 0.62933349609375 0.61566162109375 0.601806640625 0.5877685546875 0.57354736328125 0.5592041015625 0.54461669921875 0.5299072265625 0.5150146484375 0.5 0.48480224609375 0.469482421875 0.4539794921875 0.4383544921875 0.422607421875 0.40673828125 0.3907470703125 0.3746337890625 0.3583984375 0.342041015625 0.3255615234375 0.30902099609375 0.2923583984375 0.275634765625 0.2587890625 0.241943359375 0.2249755859375 0.2078857421875 0.1907958984375 0.17364501953125 0.15643310546875 0.13916015625 0.12188720703125 0.10455322265625 0.087158203125 0.06976318359375 0.05230712890625 0.034912109375 0.0174560546875 0 -0.0174560546875 -0.034912109375 -0.05230712890625 -0.06976318359375 -0.087158203125 -0.10455322265625 -0.12188720703125 -0.13916015625 -0.15643310546875 -0.17364501953125 -0.1907958984375 -0.2078857421875 -0.2249755859375 -0.241943359375 -0.2587890625 -0.275634765625 -0.2923583984375 -0.30902099609375 -0.3255615234375 -0.342041015625 -0.3583984375 -0.3746337890625 -0.3907470703125 -0.40673828125 -0.422607421875 -0.4383544921875 -0.4539794921875 -0.469482421875 -0.48480224609375 -0.5 -0.5150146484375 -0.5299072265625 -0.54461669921875 -0.5592041015625 -0.57354736328125 -0.5877685546875 -0.601806640625 -0.61566162109375 -0.62933349609375 -0.64276123046875 -0.65606689453125 -0.66912841796875 -0.6820068359375 -0.69464111328125 -0.70709228515625 -0.7193603515625 -0.7313232421875 -0.7431640625 -0.75469970703125 -0.76605224609375 -0.77716064453125 -0.78802490234375 -0.79864501953125 -0.80902099609375 -0.81915283203125 -0.82904052734375 -0.83868408203125 -0.8480224609375 -0.857177734375 -0.86602783203125 -0.8746337890625 -0.8829345703125 -0.8909912109375 -0.8988037109375 -0.90631103515625 -0.91357421875 -0.9205322265625 -0.92718505859375 -0.93359375 -0.939697265625 -0.94549560546875 -0.9510498046875 -0.956298828125 -0.96124267578125 -0.9659423828125 -0.97027587890625 -0.974365234375 -0.9781494140625 -0.98162841796875 -0.98480224609375 -0.9876708984375 -0.99029541015625 -0.9925537109375 -0.9945068359375 -0.9962158203125 -0.99755859375 -0.9986572265625 -0.9993896484375 -0.9998779296875]  VectorParams1D=off  OutDataTypeStr=fixdt(1, 16, 14)  SampleTime=-1
  HwModeRegister : Delay  DelayLength=double(1)  InitialCondition=0  SampleTime=8.33333333333333e-09
  HwModeRegister1 : Delay  DelayLength=double(1)  InitialCondition=0  SampleTime=8.33333333333333e-09
  PipelineRegister : Delay  DelayLength=double(1)  InitialCondition=0  SampleTime=8.33333333333333e-09
  Selector : Selector  NumberOfDimensions=2  IndexMode=Zero-based  SampleTime=8.33333333333333e-09  IndexOptions=Index vector (dialog),Index vector (port)  Indices=double(0),double(1)  OutputSizes=double(1),double(1)
  Selector1 : Selector  NumberOfDimensions=2  IndexMode=Zero-based  SampleTime=8.33333333333333e-09  IndexOptions=Index vector (dialog),Index vector (port)  Indices=double(0),double(1)  OutputSizes=double(1),double(1)
  delayMatch : Delay  DelayLength=double(2)  InitialCondition=0  SampleTime=8.33333333333333e-09
  xcos : Product  Inputs=**  OutDataTypeStr=fixdt(1, 25, 14)  SampleTime=8.33333333333333e-09
  xcos_in0_buff : hdlmdlgenlib/Buffer
      settings: SourceProductName=Simulink  SourceProductBaseCode=SL
  xcos_in1_buff : hdlmdlgenlib/Buffer
      settings: SourceProductName=Simulink  SourceProductBaseCode=SL
  xcos_out_dtc : DataTypeConversion  OutDataTypeStr=fixdt(1, 10, 0)  RndMeth=Round  SampleTime=8.33333333333333e-09
  Rho : Outport  VectorParamsAs1DForOutWhenUnconnected=off
  wires:
  delayMatch/1 -> Selector1/2
  Add/1 -> Rho/1
  CosineROM/1 -> Selector/1
  Selector/1 -> xcos_in1_buff/1
  Selector1/1 -> Add/2
  xcos_out_dtc/1 -> Add/1
  PipelineRegister/1 -> xcos_out_dtc/1
  X/1 -> xcos_in0_buff/1
  Y/1 -> Selector1/1
  Index/1 -> delayMatch/1, Selector/2
  xcos/1 -> PipelineRegister/1
  HwModeRegister/1 -> xcos/1
  HwModeRegister1/1 -> xcos/2
  xcos_in0_buff/1 -> HwModeRegister/1
  xcos_in1_buff/1 -> HwModeRegister1/1

== system gm_hybrid_lht/Hybrid LHT/Hybrid LHT Kernel/Gradient Kernel System/Hough Kernel/Look Ahead Hough ==
  Y : Inport  OutDataTypeStr=fixdt(1, 9, 0)  PortDimensions=1  SampleTime=8.33333333333333e-09
  eol : Inport  Port=2  OutDataTypeStr=boolean  PortDimensions=1  SampleTime=8.33333333333333e-09
  Look Ahead Hough Symmetric : Subsystem
  ysin : Outport
  wires:
  Look Ahead Hough Symmetric/1(ysin) -> ysin/1
  Y/1 -> Look Ahead Hough Symmetric/1(Y)
  eol/1 -> Look Ahead Hough Symmetric/2(eol)

== system gm_hybrid_lht/Hybrid LHT/Hybrid LHT Accumulator/Accumulator with Switches/Accumulator_instance1/Block RAM/Simple Dual Port RAM Generator ==
  wr_data : Inport  OutDataTypeStr=fixdt(0, 36, 0)  PortDimensions=1  SampleTime=8.33333333333333e-09
  wr_addr : Inport  Port=2  OutDataTypeStr=fixdt(0, 10, 0)  PortDimensions=1  SampleTime=8.33333333333333e-09
  wr_en : Inport  Port=3  OutDataTypeStr=boolean  PortDimensions=1  SampleTime=8.33333333333333e-09
  rd_addr : Inport  Port=4  OutDataTypeStr=fixdt(0, 10, 0)  PortDimensions=1  SampleTime=8.33333333333333e-09
  rd_address : hdlsllib/Logic and Bit Operations/Bit Slice  lidx=9  ridx=0
      settings: SourceProductName=Simulink  SourceProductBaseCode=SL
  simple_ram_0 : hdlsllib/HDL RAMs/Simple Dual Port RAM  ram_size=10
      settings: SourceProductName=Simulink  SourceProductBaseCode=SL
  wr_address : hdlsllib/Logic and Bit Operations/Bit Slice  lidx=9  ridx=0
      settings: SourceProductName=Simulink  SourceProductBaseCode=SL
  rd_data : Outport
  wires:
  wr_address/1 -> simple_ram_0/2
  simple_ram_0/1 -> rd_data/1
  rd_address/1 -> simple_ram_0/4
  wr_data/1 -> simple_ram_0/1
  wr_addr/1 -> wr_address/1
  wr_en/1 -> simple_ram_0/3
  rd_addr/1 -> rd_address/1

== system gm_hybrid_lht/Hybrid LHT/Hybrid LHT Accumulator/Accumulator with Switches/Accumulator_instance10/Block RAM/Simple Dual Port RAM Generator ==
  wr_data : Inport  OutDataTypeStr=fixdt(0, 36, 0)  PortDimensions=1  SampleTime=8.33333333333333e-09
  wr_addr : Inport  Port=2  OutDataTypeStr=fixdt(0, 10, 0)  PortDimensions=1  SampleTime=8.33333333333333e-09
  wr_en : Inport  Port=3  OutDataTypeStr=boolean  PortDimensions=1  SampleTime=8.33333333333333e-09
  rd_addr : Inport  Port=4  OutDataTypeStr=fixdt(0, 10, 0)  PortDimensions=1  SampleTime=8.33333333333333e-09
  rd_address : hdlsllib/Logic and Bit Operations/Bit Slice  lidx=9  ridx=0
      settings: SourceProductName=Simulink  SourceProductBaseCode=SL
  simple_ram_0 : hdlsllib/HDL RAMs/Simple Dual Port RAM  ram_size=10
      settings: SourceProductName=Simulink  SourceProductBaseCode=SL
  wr_address : hdlsllib/Logic and Bit Operations/Bit Slice  lidx=9  ridx=0
      settings: SourceProductName=Simulink  SourceProductBaseCode=SL
  rd_data : Outport
  wires:
  rd_addr/1 -> rd_address/1
  wr_en/1 -> simple_ram_0/3
  wr_addr/1 -> wr_address/1
  wr_data/1 -> simple_ram_0/1
  rd_address/1 -> simple_ram_0/4
  simple_ram_0/1 -> rd_data/1
  wr_address/1 -> simple_ram_0/2

== system gm_hybrid_lht/Hybrid LHT/Hybrid LHT Accumulator/Accumulator with Switches/Accumulator_instance11/Block RAM/Simple Dual Port RAM Generator ==
  wr_data : Inport  OutDataTypeStr=fixdt(0, 36, 0)  PortDimensions=1  SampleTime=8.33333333333333e-09
  wr_addr : Inport  Port=2  OutDataTypeStr=fixdt(0, 10, 0)  PortDimensions=1  SampleTime=8.33333333333333e-09
  wr_en : Inport  Port=3  OutDataTypeStr=boolean  PortDimensions=1  SampleTime=8.33333333333333e-09
  rd_addr : Inport  Port=4  OutDataTypeStr=fixdt(0, 10, 0)  PortDimensions=1  SampleTime=8.33333333333333e-09
  rd_address : hdlsllib/Logic and Bit Operations/Bit Slice  lidx=9  ridx=0
      settings: SourceProductName=Simulink  SourceProductBaseCode=SL
  simple_ram_0 : hdlsllib/HDL RAMs/Simple Dual Port RAM  ram_size=10
      settings: SourceProductName=Simulink  SourceProductBaseCode=SL
  wr_address : hdlsllib/Logic and Bit Operations/Bit Slice  lidx=9  ridx=0
      settings: SourceProductName=Simulink  SourceProductBaseCode=SL
  rd_data : Outport
  wires:
  rd_addr/1 -> rd_address/1
  wr_en/1 -> simple_ram_0/3
  wr_addr/1 -> wr_address/1
  wr_data/1 -> simple_ram_0/1
  rd_address/1 -> simple_ram_0/4
  simple_ram_0/1 -> rd_data/1
  wr_address/1 -> simple_ram_0/2

== system gm_hybrid_lht/Hybrid LHT/Hybrid LHT Accumulator/Accumulator with Switches/Accumulator_instance12/Block RAM/Simple Dual Port RAM Generator ==
  wr_data : Inport  OutDataTypeStr=fixdt(0, 36, 0)  PortDimensions=1  SampleTime=8.33333333333333e-09
  wr_addr : Inport  Port=2  OutDataTypeStr=fixdt(0, 10, 0)  PortDimensions=1  SampleTime=8.33333333333333e-09
  wr_en : Inport  Port=3  OutDataTypeStr=boolean  PortDimensions=1  SampleTime=8.33333333333333e-09
  rd_addr : Inport  Port=4  OutDataTypeStr=fixdt(0, 10, 0)  PortDimensions=1  SampleTime=8.33333333333333e-09
  rd_address : hdlsllib/Logic and Bit Operations/Bit Slice  lidx=9  ridx=0
      settings: SourceProductName=Simulink  SourceProductBaseCode=SL
  simple_ram_0 : hdlsllib/HDL RAMs/Simple Dual Port RAM  ram_size=10
      settings: SourceProductName=Simulink  SourceProductBaseCode=SL
  wr_address : hdlsllib/Logic and Bit Operations/Bit Slice  lidx=9  ridx=0
      settings: SourceProductName=Simulink  SourceProductBaseCode=SL
  rd_data : Outport
  wires:
  rd_addr/1 -> rd_address/1
  wr_en/1 -> simple_ram_0/3
  wr_addr/1 -> wr_address/1
  wr_data/1 -> simple_ram_0/1
  rd_address/1 -> simple_ram_0/4
  simple_ram_0/1 -> rd_data/1
  wr_address/1 -> simple_ram_0/2

== system gm_hybrid_lht/Hybrid LHT/Hybrid LHT Accumulator/Accumulator with Switches/Accumulator_instance13/Block RAM/Simple Dual Port RAM Generator ==
  wr_data : Inport  OutDataTypeStr=fixdt(0, 36, 0)  PortDimensions=1  SampleTime=8.33333333333333e-09
  wr_addr : Inport  Port=2  OutDataTypeStr=fixdt(0, 10, 0)  PortDimensions=1  SampleTime=8.33333333333333e-09
  wr_en : Inport  Port=3  OutDataTypeStr=boolean  PortDimensions=1  SampleTime=8.33333333333333e-09
  rd_addr : Inport  Port=4  OutDataTypeStr=fixdt(0, 10, 0)  PortDimensions=1  SampleTime=8.33333333333333e-09
  rd_address : hdlsllib/Logic and Bit Operations/Bit Slice  lidx=9  ridx=0
      settings: SourceProductName=Simulink  SourceProductBaseCode=SL
  simple_ram_0 : hdlsllib/HDL RAMs/Simple Dual Port RAM  ram_size=10
      settings: SourceProductName=Simulink  SourceProductBaseCode=SL
  wr_address : hdlsllib/Logic and Bit Operations/Bit Slice  lidx=9  ridx=0
      settings: SourceProductName=Simulink  SourceProductBaseCode=SL
  rd_data : Outport
  wires:
  rd_addr/1 -> rd_address/1
  wr_en/1 -> simple_ram_0/3
  wr_addr/1 -> wr_address/1
  wr_data/1 -> simple_ram_0/1
  rd_address/1 -> simple_ram_0/4
  simple_ram_0/1 -> rd_data/1
  wr_address/1 -> simple_ram_0/2

== system gm_hybrid_lht/Hybrid LHT/Hybrid LHT Accumulator/Accumulator with Switches/Accumulator_instance14/Block RAM/Simple Dual Port RAM Generator ==
  wr_data : Inport  OutDataTypeStr=fixdt(0, 36, 0)  PortDimensions=1  SampleTime=8.33333333333333e-09
  wr_addr : Inport  Port=2  OutDataTypeStr=fixdt(0, 10, 0)  PortDimensions=1  SampleTime=8.33333333333333e-09
  wr_en : Inport  Port=3  OutDataTypeStr=boolean  PortDimensions=1  SampleTime=8.33333333333333e-09
  rd_addr : Inport  Port=4  OutDataTypeStr=fixdt(0, 10, 0)  PortDimensions=1  SampleTime=8.33333333333333e-09
  rd_address : hdlsllib/Logic and Bit Operations/Bit Slice  lidx=9  ridx=0
      settings: SourceProductName=Simulink  SourceProductBaseCode=SL
  simple_ram_0 : hdlsllib/HDL RAMs/Simple Dual Port RAM  ram_size=10
      settings: SourceProductName=Simulink  SourceProductBaseCode=SL
  wr_address : hdlsllib/Logic and Bit Operations/Bit Slice  lidx=9  ridx=0
      settings: SourceProductName=Simulink  SourceProductBaseCode=SL
  rd_data : Outport
  wires:
  rd_addr/1 -> rd_address/1
  wr_en/1 -> simple_ram_0/3
  wr_addr/1 -> wr_address/1
  wr_data/1 -> simple_ram_0/1
  rd_address/1 -> simple_ram_0/4
  simple_ram_0/1 -> rd_data/1
  wr_address/1 -> simple_ram_0/2

== system gm_hybrid_lht/Hybrid LHT/Hybrid LHT Accumulator/Accumulator with Switches/Accumulator_instance15/Block RAM/Simple Dual Port RAM Generator ==
  wr_data : Inport  OutDataTypeStr=fixdt(0, 36, 0)  PortDimensions=1  SampleTime=8.33333333333333e-09
  wr_addr : Inport  Port=2  OutDataTypeStr=fixdt(0, 10, 0)  PortDimensions=1  SampleTime=8.33333333333333e-09
  wr_en : Inport  Port=3  OutDataTypeStr=boolean  PortDimensions=1  SampleTime=8.33333333333333e-09
  rd_addr : Inport  Port=4  OutDataTypeStr=fixdt(0, 10, 0)  PortDimensions=1  SampleTime=8.33333333333333e-09
  rd_address : hdlsllib/Logic and Bit Operations/Bit Slice  lidx=9  ridx=0
      settings: SourceProductName=Simulink  SourceProductBaseCode=SL
  simple_ram_0 : hdlsllib/HDL RAMs/Simple Dual Port RAM  ram_size=10
      settings: SourceProductName=Simulink  SourceProductBaseCode=SL
  wr_address : hdlsllib/Logic and Bit Operations/Bit Slice  lidx=9  ridx=0
      settings: SourceProductName=Simulink  SourceProductBaseCode=SL
  rd_data : Outport
  wires:
  rd_addr/1 -> rd_address/1
  wr_en/1 -> simple_ram_0/3
  wr_addr/1 -> wr_address/1
  wr_data/1 -> simple_ram_0/1
  rd_address/1 -> simple_ram_0/4
  simple_ram_0/1 -> rd_data/1
  wr_address/1 -> simple_ram_0/2

== system gm_hybrid_lht/Hybrid LHT/Hybrid LHT Accumulator/Accumulator with Switches/Accumulator_instance16/Block RAM/Simple Dual Port RAM Generator ==
  wr_data : Inport  OutDataTypeStr=fixdt(0, 36, 0)  PortDimensions=1  SampleTime=8.33333333333333e-09
  wr_addr : Inport  Port=2  OutDataTypeStr=fixdt(0, 10, 0)  PortDimensions=1  SampleTime=8.33333333333333e-09
  wr_en : Inport  Port=3  OutDataTypeStr=boolean  PortDimensions=1  SampleTime=8.33333333333333e-09
  rd_addr : Inport  Port=4  OutDataTypeStr=fixdt(0, 10, 0)  PortDimensions=1  SampleTime=8.33333333333333e-09
  rd_address : hdlsllib/Logic and Bit Operations/Bit Slice  lidx=9  ridx=0
      settings: SourceProductName=Simulink  SourceProductBaseCode=SL
  simple_ram_0 : hdlsllib/HDL RAMs/Simple Dual Port RAM  ram_size=10
      settings: SourceProductName=Simulink  SourceProductBaseCode=SL
  wr_address : hdlsllib/Logic and Bit Operations/Bit Slice  lidx=9  ridx=0
      settings: SourceProductName=Simulink  SourceProductBaseCode=SL
  rd_data : Outport
  wires:
  rd_addr/1 -> rd_address/1
  wr_en/1 -> simple_ram_0/3
  wr_addr/1 -> wr_address/1
  wr_data/1 -> simple_ram_0/1
  rd_address/1 -> simple_ram_0/4
  simple_ram_0/1 -> rd_data/1
  wr_address/1 -> simple_ram_0/2

== system gm_hybrid_lht/Hybrid LHT/Hybrid LHT Accumulator/Accumulator with Switches/Accumulator_instance17/Block RAM/Simple Dual Port RAM Generator ==
  wr_data : Inport  OutDataTypeStr=fixdt(0, 36, 0)  PortDimensions=1  SampleTime=8.33333333333333e-09
  wr_addr : Inport  Port=2  OutDataTypeStr=fixdt(0, 10, 0)  PortDimensions=1  SampleTime=8.33333333333333e-09
  wr_en : Inport  Port=3  OutDataTypeStr=boolean  PortDimensions=1  SampleTime=8.33333333333333e-09
  rd_addr : Inport  Port=4  OutDataTypeStr=fixdt(0, 10, 0)  PortDimensions=1  SampleTime=8.33333333333333e-09
  rd_address : hdlsllib/Logic and Bit Operations/Bit Slice  lidx=9  ridx=0
      settings: SourceProductName=Simulink  SourceProductBaseCode=SL
  simple_ram_0 : hdlsllib/HDL RAMs/Simple Dual Port RAM  ram_size=10
      settings: SourceProductName=Simulink  SourceProductBaseCode=SL
  wr_address : hdlsllib/Logic and Bit Operations/Bit Slice  lidx=9  ridx=0
      settings: SourceProductName=Simulink  SourceProductBaseCode=SL
  rd_data : Outport
  wires:
  rd_addr/1 -> rd_address/1
  wr_en/1 -> simple_ram_0/3
  wr_addr/1 -> wr_address/1
  wr_data/1 -> simple_ram_0/1
  rd_address/1 -> simple_ram_0/4
  simple_ram_0/1 -> rd_data/1
  wr_address/1 -> simple_ram_0/2
